simulink model "vi_du_2"  (R2015a)
settings: Solver=ode4  SolverMode=SingleTasking  StartTime=0.0  StopTime=80  FixedStep=0.001  RelTol=1e-3
settings Model: CovMetricSettings=dwe  CovHtmlReporting=off  covSaveCumulativeToWorkspaceVar=off  CovSaveSingleToWorkspaceVar=off  CovExternalEMLEnable=on  Creator=ryell  LastModifiedBy=ryell
settings DataIOCC: LimitDataPoints=off  SaveFormat=Dataset
settings DebuggingCC: SFUnexpectedBacktrackingDiag=error  SFNoUnconditionalDefaultTransitionDiag=error
settings HardwareCC: ProdBitPerPointer=64  ProdLargestAtomicFloat=Float  ProdIntDivRoundTo=Zero  ProdEndianess=LittleEndian  ProdHWDeviceType=Specified
settings ModelReferenceCC: PropagateSignalLabelsOutOfModel=on
settings GRTTargetCC: TargetLangStandard=C99 (ISO)  GeneratePreprocessorConditionals=Use local settings

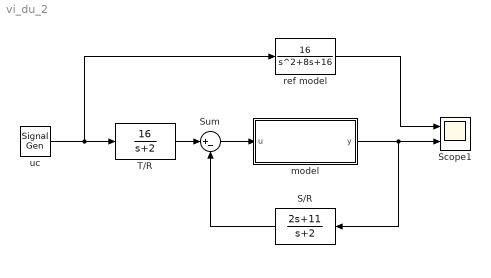
== system vi_du_2 ==
  S/R : TransferFcn  Numerator=[2 11]  Denominator=[1 2]
  Scope1 : Scope  NumInputPorts=2
      settings: TimeRange=auto  ShowLegends=on  MaxDataPoints=5000  SaveToWorkspace=off  YMin=-1.5~-5  YMax=1.5~5  SampleTime=-1
  Sum : Sum  Inputs=|+-
  T/R : TransferFcn  Numerator=[16]  Denominator=[1 2]
  model : Subsystem
  ref model : TransferFcn  Numerator=[16]  Denominator=[1 8 16]
  uc : SignalGenerator  WaveForm=square  Frequency=0.1
  wires:
  uc/1 -> ref model/1, T/R/1
  T/R/1 -> Sum/1
  model/1(y) -> Scope1/2, S/R/1
  S/R/1 -> Sum/2
  ref model/1 -> Scope1/1
  Sum/1 -> model/1(u)

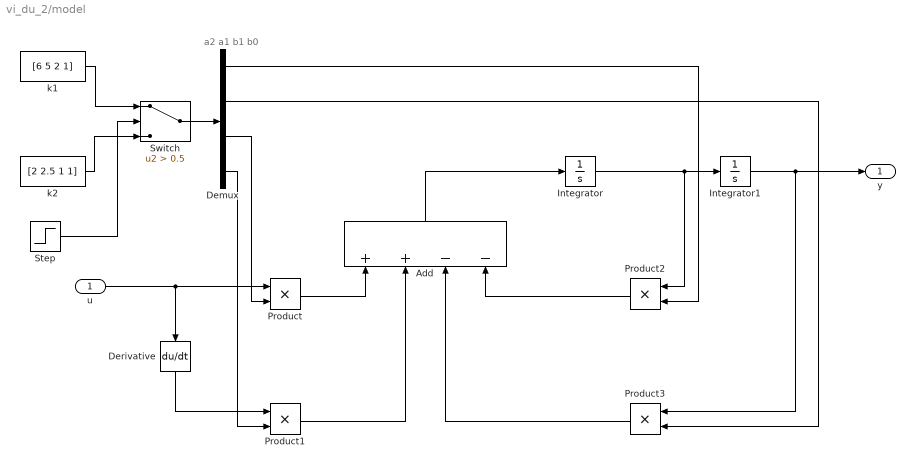
== system vi_du_2/model ==
  note: a2 a1 b1 b0
  u : Inport
  Add : Sum  Inputs=++--
  Demux : Demux
  Derivative : Derivative
  Integrator : Integrator
  Integrator1 : Integrator
  Product{,1..3} (4 alike) : Product
  Step : Step  Time=40  Before=1  After=0  SampleTime=0
  Switch : Switch  Criteria=u2 > Threshold  Threshold=0.5
  k1 : Constant  Value=[6 5 2 1]
  k2 : Constant  Value=[2 2.5 1 1]
  y : Outport
  wires:
  Product/1 -> Add/1
  Product1/1 -> Add/2
  Derivative/1 -> Product1/1
  u/1 -> Derivative/1, Product/1
  Add/1 -> Integrator/1
  Integrator/1 -> Product2/1, Integrator1/1
  Integrator1/1 -> Product3/1, y/1
  Product3/1 -> Add/3
  Product2/1 -> Add/4
  Switch/1 -> Demux/1
  k1/1 -> Switch/1
  k2/1 -> Switch/3
  Demux/4 -> Product1/2
  Demux/3 -> Product/2
  Demux/1 -> Product2/2
  Step/1 -> Switch/2
  Demux/2 -> Product3/2
